simulink model "ARINC429_DW"  (R2020b)
settings: Solver=VariableStepAuto  StartTime=0.0  StopTime=10.0  RelTol=1e-3
(part 1 of 2)
settings Model: Creator=Nicolas  LastModifiedBy=rolla

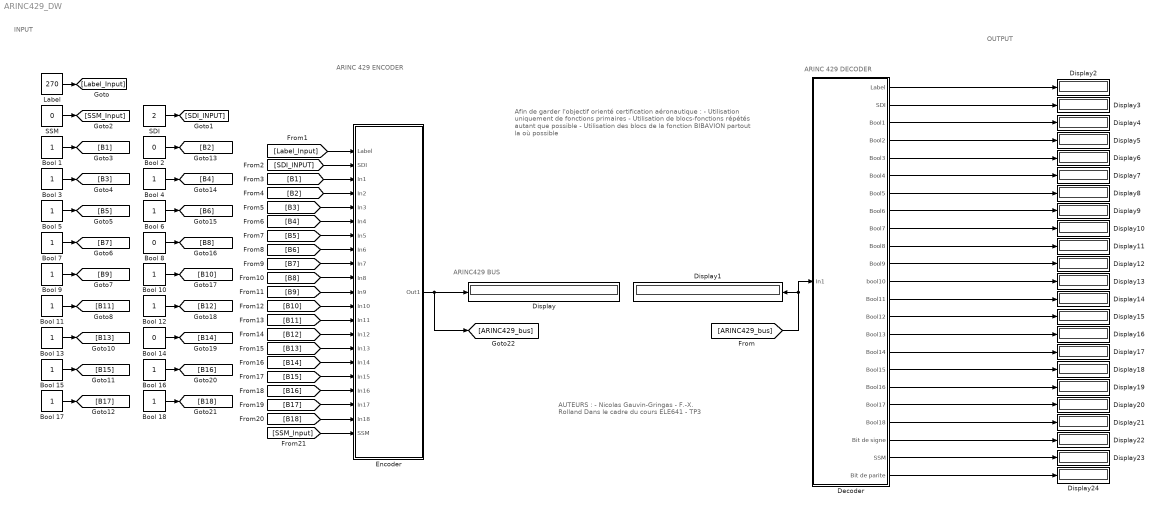
== system ARINC429_DW ==
  note: ARINC 429 DECODER
  note: ARINC 429 ENCODER
  note: ARINC429 BUS
  note: OUTPUT
  note: INPUT
  note: AUTEURS :
      | - Nicolas Gauvin-Gringas
      | - F.-X. Rolland
      |
      | Dans le cadre du cours ELE641 - TP3
  note: Afin de garder l'objectif orienté certification aéronautique :
      | - Utilisation uniquement de fonctions primaires
      | - Utilisation de blocs-fonctions répétés autant que possible
      | - Utilisation des blocs de la fonction BIBAVION partout la où possible
  Bool {1,3..7,9..13,15..18} (15 alike) : Constant  OutDataTypeStr=boolean
  Bool 14 : Constant  Value=0  OutDataTypeStr=boolean
  Bool 2 : Constant  Value=0  OutDataTypeStr=boolean
  Bool 8 : Constant  Value=0  OutDataTypeStr=boolean
  Decoder : Subsystem
  Display{,1..24} (25 alike) : Display
      Display settings: Format=binary (Stored Integer)
      Display1 settings: Format=binary (Stored Integer)
  Encoder : Subsystem
  Label : Constant  Value=270  OutDataTypeStr=uint32  SampleTime=-1
  SDI : Constant  Value=2  OutDataTypeStr=uint32  SampleTime=-1
  SSM : Constant  Value=0  OutDataTypeStr=uint32  SampleTime=-1
  wires:
  [ARINC429_bus] -> Decoder/1(In1), Display1/1
  Label/1 -> [Label_Input]
  SDI/1 -> [SDI_INPUT]
  SSM/1 -> [SSM_Input]
  Decoder/1(Label) -> Display2/1
  Bool 1/1 -> [B1]
  Bool 2/1 -> [B2]
  Bool 18/1 -> [B18]
  Bool 16/1 -> [B16]
  Bool 14/1 -> [B14]
  Bool 12/1 -> [B12]
  Bool 10/1 -> [B10]
  Bool 8/1 -> [B8]
  Bool 6/1 -> [B6]
  Bool 4/1 -> [B4]
  Bool 3/1 -> [B3]
  Bool 5/1 -> [B5]
  Bool 7/1 -> [B7]
  Bool 9/1 -> [B9]
  Bool 11/1 -> [B11]
  Bool 13/1 -> [B13]
  Bool 15/1 -> [B15]
  Bool 17/1 -> [B17]
  [Label_Input] -> Encoder/1(Label)
  Encoder/1(Out1) -> [ARINC429_bus], Display/1
  [SDI_INPUT] -> Encoder/2(SDI)
  [B1] -> Encoder/3(In1)
  [B2] -> Encoder/4(In2)
  [B3] -> Encoder/5(In3)
  [B4] -> Encoder/6(In4)
  [B5] -> Encoder/7(In5)
  [B6] -> Encoder/8(In6)
  [B7] -> Encoder/9(In7)
  [B8] -> Encoder/10(In8)
  [B9] -> Encoder/11(In9)
  [B10] -> Encoder/12(In10)
  [B11] -> Encoder/13(In11)
  [B12] -> Encoder/14(In12)
  [B13] -> Encoder/15(In13)
  [B14] -> Encoder/16(In14)
  [B15] -> Encoder/17(In15)
  [B16] -> Encoder/18(In16)
  [B17] -> Encoder/19(In17)
  [B18] -> Encoder/20(In18)
  [SSM_Input] -> Encoder/21(SSM)
  Decoder/2(SDI) -> Display3/1
  Decoder/3(Bool1) -> Display4/1
  Decoder/4(Bool2) -> Display5/1
  Decoder/5(Bool3) -> Display6/1
  Decoder/6(Bool4) -> Display7/1
  Decoder/7(Bool5) -> Display8/1
  Decoder/8(Bool6) -> Display9/1
  Decoder/9(Bool7) -> Display10/1
  Decoder/10(Bool8) -> Display11/1
  Decoder/11(Bool9) -> Display12/1
  Decoder/12(bool10) -> Display13/1
  Decoder/13(Bool11) -> Display14/1
  Decoder/14(Bool12) -> Display15/1
  Decoder/15(Bool13) -> Display16/1
  Decoder/16(Bool14) -> Display17/1
  Decoder/17(Bool15) -> Display18/1
  Decoder/18(Bool16) -> Display19/1
  Decoder/19(Bool17) -> Display20/1
  Decoder/20(Bool18) -> Display21/1
  Decoder/21(Bit de signe) -> Display22/1
  Decoder/22(SSM) -> Display23/1
  Decoder/23(Bit de parite) -> Display24/1

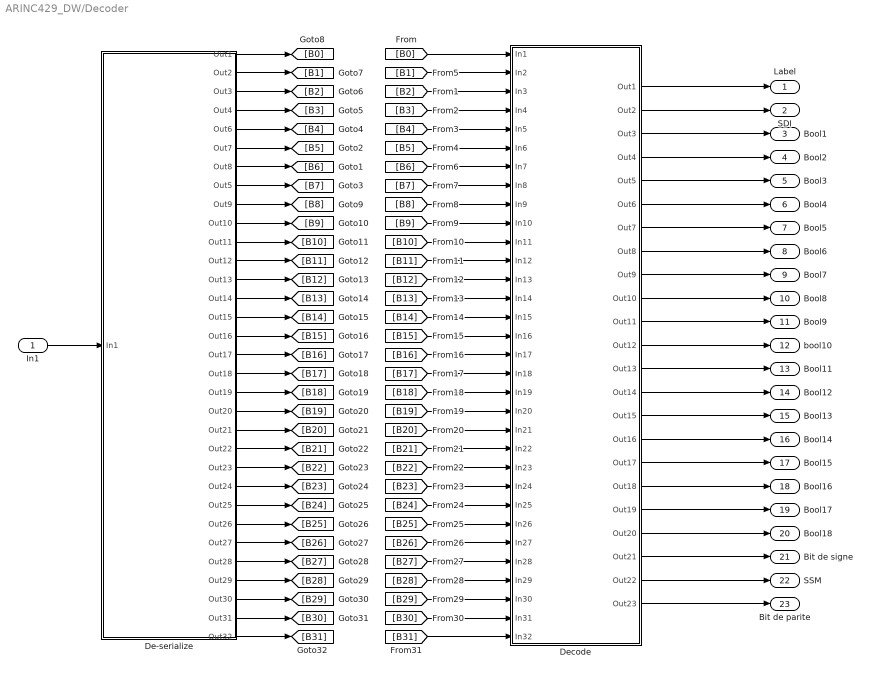
== system ARINC429_DW/Decoder ==
  In1 : Inport
  De-serialize : Subsystem
  Decode : Subsystem
  Label : Outport
  SDI : Outport  Port=2
  Bool1 : Outport  Port=3
  Bool2 : Outport  Port=4
  Bool3 : Outport  Port=5
  Bool4 : Outport  Port=6
  Bool5 : Outport  Port=7
  Bool6 : Outport  Port=8
  Bool7 : Outport  Port=9
  Bool8 : Outport  Port=10
  Bool9 : Outport  Port=11
  bool10 : Outport  Port=12
  Bool11 : Outport  Port=13
  Bool12 : Outport  Port=14
  Bool13 : Outport  Port=15
  Bool14 : Outport  Port=16
  Bool15 : Outport  Port=17
  Bool16 : Outport  Port=18
  Bool17 : Outport  Port=19
  Bool18 : Outport  Port=20
  Bit de signe : Outport  Port=21
  SSM : Outport  Port=22
  Bit de parite : Outport  Port=23
  wires:
  De-serialize/6(Out7) -> [B5]
  De-serialize/1(Out1) -> [B0]
  De-serialize/7(Out8) -> [B6]
  De-serialize/5(Out6) -> [B4]
  De-serialize/3(Out3) -> [B2]
  De-serialize/2(Out2) -> [B1]
  De-serialize/4(Out4) -> [B3]
  De-serialize/8(Out5) -> [B7]
  In1/1 -> De-serialize/1(In1)
  [B1] -> Decode/2(In2)
  [B0] -> Decode/1(In1)
  [B2] -> Decode/3(In3)
  [B3] -> Decode/4(In4)
  [B4] -> Decode/5(In5)
  [B5] -> Decode/6(In6)
  [B6] -> Decode/7(In7)
  [B7] -> Decode/8(In8)
  Decode/1(Out1) -> Label/1
  De-serialize/9(Out9) -> [B8]
  De-serialize/10(Out10) -> [B9]
  De-serialize/11(Out11) -> [B10]
  De-serialize/12(Out12) -> [B11]
  De-serialize/13(Out13) -> [B12]
  De-serialize/14(Out14) -> [B13]
  De-serialize/15(Out15) -> [B14]
  De-serialize/16(Out16) -> [B15]
  De-serialize/17(Out17) -> [B16]
  De-serialize/18(Out18) -> [B17]
  De-serialize/19(Out19) -> [B18]
  De-serialize/20(Out20) -> [B19]
  De-serialize/21(Out21) -> [B20]
  De-serialize/22(Out22) -> [B21]
  De-serialize/23(Out23) -> [B22]
  De-serialize/24(Out24) -> [B23]
  De-serialize/25(Out25) -> [B24]
  De-serialize/26(Out26) -> [B25]
  De-serialize/27(Out27) -> [B26]
  De-serialize/28(Out28) -> [B27]
  De-serialize/29(Out29) -> [B28]
  De-serialize/30(Out30) -> [B29]
  De-serialize/31(Out31) -> [B30]
  De-serialize/32(Out32) -> [B31]
  [B8] -> Decode/9(In9)
  [B9] -> Decode/10(In10)
  [B10] -> Decode/11(In11)
  [B11] -> Decode/12(In12)
  [B12] -> Decode/13(In13)
  [B13] -> Decode/14(In14)
  [B14] -> Decode/15(In15)
  [B15] -> Decode/16(In16)
  [B16] -> Decode/17(In17)
  [B17] -> Decode/18(In18)
  [B18] -> Decode/19(In19)
  [B19] -> Decode/20(In20)
  [B20] -> Decode/21(In21)
  [B21] -> Decode/22(In22)
  [B22] -> Decode/23(In23)
  [B23] -> Decode/24(In24)
  [B24] -> Decode/25(In25)
  [B25] -> Decode/26(In26)
  [B26] -> Decode/27(In27)
  [B27] -> Decode/28(In28)
  [B28] -> Decode/29(In29)
  [B29] -> Decode/30(In30)
  [B30] -> Decode/31(In31)
  [B31] -> Decode/32(In32)
  Decode/3(Out3) -> Bool1/1
  Decode/4(Out4) -> Bool2/1
  Decode/5(Out5) -> Bool3/1
  Decode/10(Out10) -> Bool8/1
  Decode/11(Out11) -> Bool9/1
  Decode/12(Out12) -> bool10/1
  Decode/13(Out13) -> Bool11/1
  Decode/14(Out14) -> Bool12/1
  Decode/15(Out15) -> Bool13/1
  Decode/16(Out16) -> Bool14/1
  Decode/17(Out17) -> Bool15/1
  Decode/18(Out18) -> Bool16/1
  Decode/19(Out19) -> Bool17/1
  Decode/20(Out20) -> Bool18/1
  Decode/21(Out21) -> Bit de signe/1
  Decode/22(Out22) -> SSM/1
  Decode/23(Out23) -> Bit de parite/1
  Decode/9(Out9) -> Bool7/1
  Decode/8(Out8) -> Bool6/1
  Decode/7(Out7) -> Bool5/1
  Decode/6(Out6) -> Bool4/1
  Decode/2(Out2) -> SDI/1

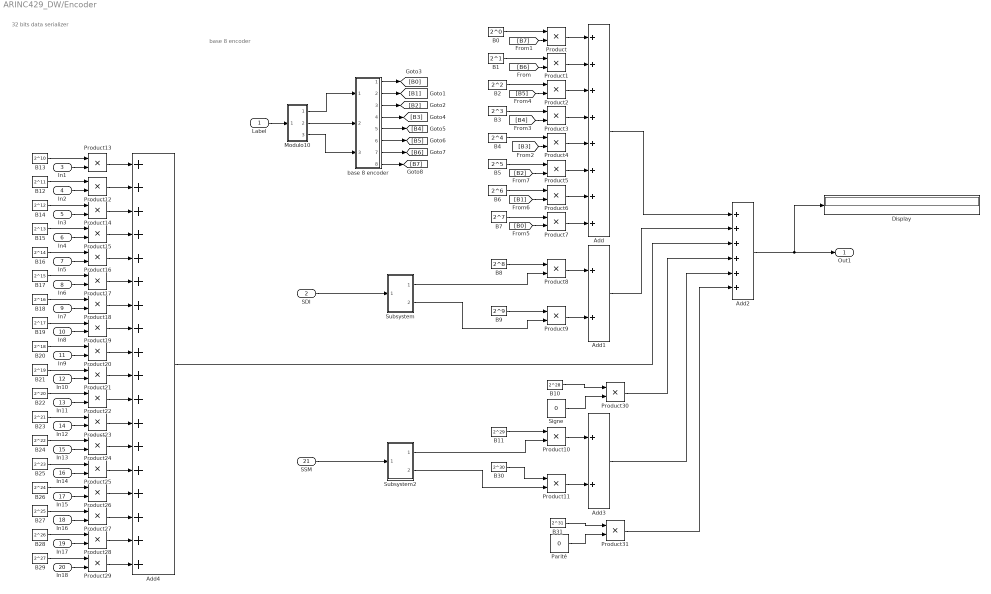
== system ARINC429_DW/Encoder ==
  note: base 8 encoder
  note: 32 bits data serializer
  Label : Inport
  SDI : Inport  Port=2
  In1 : Inport  Port=3
  In2 : Inport  Port=4
  In3 : Inport  Port=5
  In4 : Inport  Port=6
  In5 : Inport  Port=7
  In6 : Inport  Port=8
  In7 : Inport  Port=9
  In8 : Inport  Port=10
  In9 : Inport  Port=11
  In10 : Inport  Port=12
  In11 : Inport  Port=13
  In12 : Inport  Port=14
  In13 : Inport  Port=15
  In14 : Inport  Port=16
  In15 : Inport  Port=17
  In16 : Inport  Port=18
  In17 : Inport  Port=19
  In18 : Inport  Port=20
  SSM : Inport  Port=21
  Add : Sum  Inputs=++++++++  AccumDataTypeStr=uint32  OutDataTypeStr=uint32
  Add1 : Sum
  Add2 : Sum  Inputs=++++++  AccumDataTypeStr=uint32  OutDataTypeStr=uint32
  Add3 : Sum
  Add4 : Sum  Inputs=++++++++++++++++++
  B0 : Constant  Value=2^0  OutDataTypeStr=single
  B1 : Constant  Value=2^1  OutDataTypeStr=single
  B10 : Constant  Value=2^28  OutDataTypeStr=single
  B11 : Constant  Value=2^29  OutDataTypeStr=single
  B12 : Constant  Value=2^11  OutDataTypeStr=single
  B13 : Constant  Value=2^10  OutDataTypeStr=single
  B14 : Constant  Value=2^12  OutDataTypeStr=single
  B15 : Constant  Value=2^13  OutDataTypeStr=single
  B16 : Constant  Value=2^14  OutDataTypeStr=single
  B17 : Constant  Value=2^15  OutDataTypeStr=single
  B18 : Constant  Value=2^16  OutDataTypeStr=single
  B19 : Constant  Value=2^17  OutDataTypeStr=single
  B2 : Constant  Value=2^2  OutDataTypeStr=single
  B20 : Constant  Value=2^18  OutDataTypeStr=single
  B21 : Constant  Value=2^19  OutDataTypeStr=single
  B22 : Constant  Value=2^20  OutDataTypeStr=single
  B23 : Constant  Value=2^21  OutDataTypeStr=single
  B24 : Constant  Value=2^22  OutDataTypeStr=single
  B25 : Constant  Value=2^23  OutDataTypeStr=single
  B26 : Constant  Value=2^24  OutDataTypeStr=single
  B27 : Constant  Value=2^25  OutDataTypeStr=single
  B28 : Constant  Value=2^26  OutDataTypeStr=single
  B29 : Constant  Value=2^27  OutDataTypeStr=single
  B3 : Constant  Value=2^3  OutDataTypeStr=single
  B30 : Constant  Value=2^30  OutDataTypeStr=single
  B31 : Constant  Value=2^31  OutDataTypeStr=single
  B4 : Constant  Value=2^4  OutDataTypeStr=single
  B5 : Constant  Value=2^5  OutDataTypeStr=single
  B6 : Constant  Value=2^6  OutDataTypeStr=single
  B7 : Constant  Value=2^7  OutDataTypeStr=single
  B8 : Constant  Value=2^8  OutDataTypeStr=single
  B9 : Constant  Value=2^9  OutDataTypeStr=single
  Display : Display
      settings: Format=binary (Stored Integer)
  "Modulo10 " : Subsystem
  Parité : Constant  Value=0  OutDataTypeStr=boolean
  Product{,1..31} (32 alike) : Product
  Signe : Constant  Value=0  OutDataTypeStr=boolean
  Subsystem : Subsystem
  Subsystem2 : Subsystem
  base 8 encoder : Subsystem
  Out1 : Outport
  wires:
  base 8 encoder/4(Out4) -> [B3]
  B5/1 -> Product5/1
  [B0] -> Product7/2
  B2/1 -> Product2/1
  [B5] -> Product2/2
  [B3] -> Product4/2
  "Modulo10 "/2(Out2) -> base 8 encoder/2(In2)
  "Modulo10 "/3(Out3) -> base 8 encoder/3(In3)
  B0/1 -> Product/1
  Product3/1 -> Add/4
  [B7] -> Product/2
  Product4/1 -> Add/5
  base 8 encoder/5(Out5) -> [B4]
  base 8 encoder/8(Out8) -> [B7]
  [B6] -> Product1/2
  B1/1 -> Product1/1
  [B4] -> Product3/2
  B4/1 -> Product4/1
  base 8 encoder/3(Out3) -> [B2]
  Product/1 -> Add/1
  Product5/1 -> Add/6
  Product6/1 -> Add/7
  base 8 encoder/1(Out1) -> [B0]
  [B1] -> Product6/2
  base 8 encoder/7(Out7) -> [B6]
  Product2/1 -> Add/3
  B3/1 -> Product3/1
  Label/1 -> "Modulo10 "/1(In1)
  Product7/1 -> Add/8
  Product1/1 -> Add/2
  B6/1 -> Product6/1
  B7/1 -> Product7/1
  "Modulo10 "/1(Out1) -> base 8 encoder/1(In1)
  base 8 encoder/6(Out6) -> [B5]
  [B2] -> Product5/2
  base 8 encoder/2(Out2) -> [B1]
  Product9/1 -> Add1/2
  Product8/1 -> Add1/1
  B9/1 -> Product9/1
  B8/1 -> Product8/1
  Product10/1 -> Add3/1
  Product11/1 -> Add3/2
  B13/1 -> Product13/1
  Product13/1 -> Add4/1
  B12/1 -> Product12/1
  Product12/1 -> Add4/2
  B14/1 -> Product14/1
  Product14/1 -> Add4/3
  B15/1 -> Product15/1
  Product15/1 -> Add4/4
  B16/1 -> Product16/1
  Product16/1 -> Add4/5
  B17/1 -> Product17/1
  Product17/1 -> Add4/6
  B18/1 -> Product18/1
  Product18/1 -> Add4/7
  B19/1 -> Product19/1
  Product19/1 -> Add4/8
  B20/1 -> Product20/1
  Product20/1 -> Add4/9
  B21/1 -> Product21/1
  Product21/1 -> Add4/10
  B22/1 -> Product22/1
  Product22/1 -> Add4/11
  B23/1 -> Product23/1
  Product23/1 -> Add4/12
  B24/1 -> Product24/1
  Product24/1 -> Add4/13
  B25/1 -> Product25/1
  Product25/1 -> Add4/14
  B26/1 -> Product26/1
  Product26/1 -> Add4/15
  B27/1 -> Product27/1
  Product27/1 -> Add4/16
  B28/1 -> Product28/1
  Product28/1 -> Add4/17
  B29/1 -> Product29/1
  Product29/1 -> Add4/18
  In1/1 -> Product13/2
  In2/1 -> Product12/2
  In3/1 -> Product14/2
  In4/1 -> Product15/2
  In5/1 -> Product16/2
  In6/1 -> Product17/2
  In7/1 -> Product18/2
  In8/1 -> Product19/2
  In9/1 -> Product20/2
  In10/1 -> Product21/2
  In11/1 -> Product22/2
  In12/1 -> Product23/2
  In13/1 -> Product24/2
  In14/1 -> Product25/2
  In15/1 -> Product26/2
  In16/1 -> Product27/2
  In17/1 -> Product28/2
  In18/1 -> Product29/2
  SDI/1 -> Subsystem/1(In1)
  Subsystem/1(Out1) -> Product8/2
  Subsystem/2(Out2) -> Product9/2
  SSM/1 -> Subsystem2/1(In1)
  Subsystem2/1(Out1) -> Product10/2
  Subsystem2/2(Out2) -> Product11/2
  Signe/1 -> Product30/2
  B31/1 -> Product31/1
  Parité/1 -> Product31/2
  B11/1 -> Product10/1
  B10/1 -> Product30/1
  Add2/1 -> Display/1, Out1/1
  Add/1 -> Add2/1
  Add1/1 -> Add2/2
  Add4/1 -> Add2/3
  Product30/1 -> Add2/4
  Add3/1 -> Add2/5
  Product31/1 -> Add2/6
  B30/1 -> Product11/1

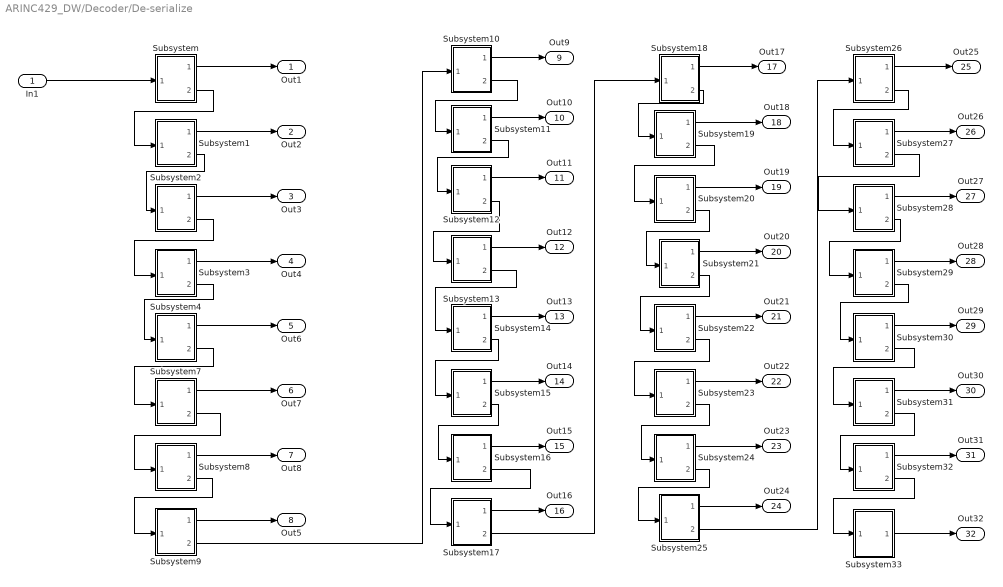
== system ARINC429_DW/Decoder/De-serialize ==
  In1 : Inport
  Subsystem : Subsystem
  Subsystem1 : Subsystem
  Subsystem10 : Subsystem
  Subsystem11 : Subsystem
  Subsystem12 : Subsystem
  Subsystem13 : Subsystem
  Subsystem14 : Subsystem
  Subsystem15 : Subsystem
  Subsystem16 : Subsystem
  Subsystem17 : Subsystem
  Subsystem18 : Subsystem
  Subsystem19 : Subsystem
  Subsystem2 : Subsystem
  Subsystem20 : Subsystem
  Subsystem21 : Subsystem
  Subsystem22 : Subsystem
  Subsystem23 : Subsystem
  Subsystem24 : Subsystem
  Subsystem25 : Subsystem
  Subsystem26 : Subsystem
  Subsystem27 : Subsystem
  Subsystem28 : Subsystem
  Subsystem29 : Subsystem
  Subsystem3 : Subsystem
  Subsystem30 : Subsystem
  Subsystem31 : Subsystem
  Subsystem32 : Subsystem
  Subsystem33 : Subsystem
  Subsystem4 : Subsystem
  Subsystem7 : Subsystem
  Subsystem8 : Subsystem
  Subsystem9 : Subsystem
  Out1 : Outport
  Out2 : Outport  Port=2
  Out3 : Outport  Port=3
  Out4 : Outport  Port=4
  Out6 : Outport  Port=5
  Out7 : Outport  Port=6
  Out8 : Outport  Port=7
  Out5 : Outport  Port=8
  Out9 : Outport  Port=9
  Out10 : Outport  Port=10
  Out11 : Outport  Port=11
  Out12 : Outport  Port=12
  Out13 : Outport  Port=13
  Out14 : Outport  Port=14
  Out15 : Outport  Port=15
  Out16 : Outport  Port=16
  Out17 : Outport  Port=17
  Out18 : Outport  Port=18
  Out19 : Outport  Port=19
  Out20 : Outport  Port=20
  Out21 : Outport  Port=21
  Out22 : Outport  Port=22
  Out23 : Outport  Port=23
  Out24 : Outport  Port=24
  Out25 : Outport  Port=25
  Out26 : Outport  Port=26
  Out27 : Outport  Port=27
  Out28 : Outport  Port=28
  Out29 : Outport  Port=29
  Out30 : Outport  Port=30
  Out31 : Outport  Port=31
  Out32 : Outport  Port=32
  wires:
  Subsystem/1(Out1) -> Out1/1
  Subsystem1/1(Out1) -> Out2/1
  Subsystem1/2(Out2) -> Subsystem2/1(In1)
  Subsystem2/2(Out2) -> Subsystem3/1(In1)
  Subsystem3/2(Out2) -> Subsystem4/1(In1)
  Subsystem2/1(Out1) -> Out3/1
  Subsystem3/1(Out1) -> Out4/1
  Subsystem4/2(Out2) -> Subsystem7/1(In1)
  Subsystem4/1(Out1) -> Out6/1
  Subsystem7/1(Out1) -> Out7/1
  Subsystem8/1(Out1) -> Out8/1
  Subsystem10/2(Out2) -> Subsystem11/1(In1)
  Subsystem12/2(Out2) -> Subsystem13/1(In1)
  Subsystem14/2(Out2) -> Subsystem15/1(In1)
  Subsystem11/2(Out2) -> Subsystem12/1(In1)
  Subsystem15/2(Out2) -> Subsystem16/1(In1)
  Subsystem16/2(Out2) -> Subsystem17/1(In1)
  Subsystem23/2(Out2) -> Subsystem24/1(In1)
  Subsystem18/2(Out2) -> Subsystem19/1(In1)
  Subsystem21/2(Out2) -> Subsystem22/1(In1)
  Subsystem22/2(Out2) -> Subsystem23/1(In1)
  Subsystem19/2(Out2) -> Subsystem20/1(In1)
  Subsystem20/2(Out2) -> Subsystem21/1(In1)
  Subsystem24/2(Out2) -> Subsystem25/1(In1)
  Subsystem29/2(Out2) -> Subsystem30/1(In1)
  Subsystem27/2(Out2) -> Subsystem28/1(In1)
  Subsystem28/2(Out2) -> Subsystem29/1(In1)
  Subsystem26/2(Out2) -> Subsystem27/1(In1)
  Subsystem9/1(Out1) -> Out5/1
  Subsystem17/2(Out2) -> Subsystem18/1(In1)
  Subsystem25/2(Out2) -> Subsystem26/1(In1)
  Subsystem9/2(Out2) -> Subsystem10/1(In1)
  Subsystem10/1(Out1) -> Out9/1
  Subsystem11/1(Out1) -> Out10/1
  Subsystem12/1(Out1) -> Out11/1
  Subsystem13/1(Out1) -> Out12/1
  Subsystem14/1(Out1) -> Out13/1
  Subsystem15/1(Out1) -> Out14/1
  Subsystem16/1(Out1) -> Out15/1
  Subsystem17/1(Out1) -> Out16/1
  Subsystem18/1(Out1) -> Out17/1
  Subsystem19/1(Out1) -> Out18/1
  Subsystem20/1(Out1) -> Out19/1
  Subsystem21/1(Out1) -> Out20/1
  Subsystem22/1(Out1) -> Out21/1
  Subsystem23/1(Out1) -> Out22/1
  Subsystem24/1(Out1) -> Out23/1
  Subsystem25/1(Out1) -> Out24/1
  Subsystem26/1(Out1) -> Out25/1
  Subsystem27/1(Out1) -> Out26/1
  Subsystem28/1(Out1) -> Out27/1
  Subsystem29/1(Out1) -> Out28/1
  Subsystem33/1(Out1) -> Out32/1
  Subsystem30/2(Out2) -> Subsystem31/1(In1)
  Subsystem31/2(Out2) -> Subsystem32/1(In1)
  Subsystem32/2(Out2) -> Subsystem33/1(In1)
  Subsystem32/1(Out1) -> Out31/1
  Subsystem31/1(Out1) -> Out30/1
  Subsystem30/1(Out1) -> Out29/1
  Subsystem7/2(Out2) -> Subsystem8/1(In1)
  Subsystem8/2(Out2) -> Subsystem9/1(In1)
  Subsystem/2(Out2) -> Subsystem1/1(In1)
  In1/1 -> Subsystem/1(In1)
  Subsystem13/2(Out2) -> Subsystem14/1(In1)

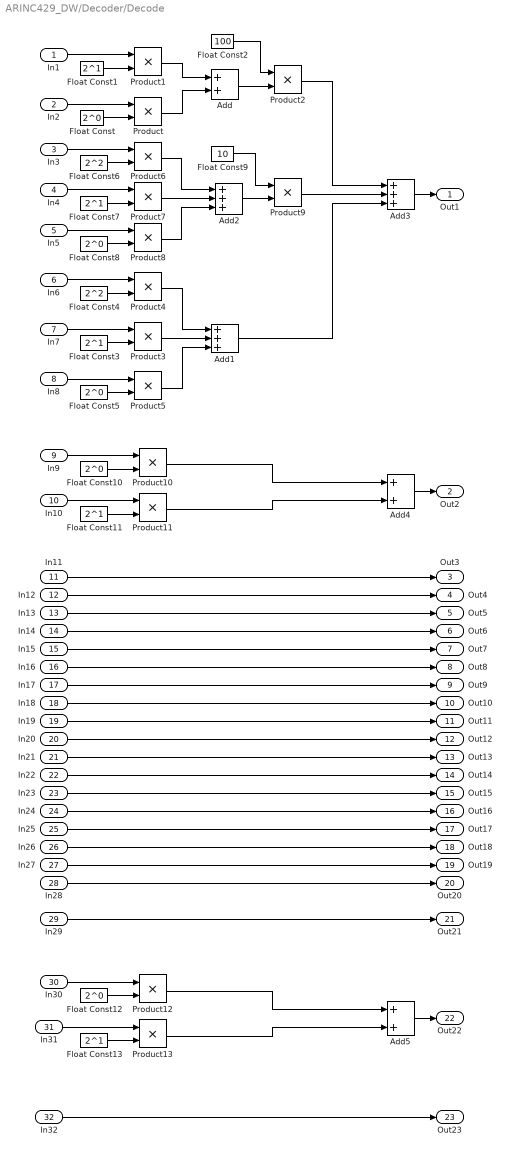
== system ARINC429_DW/Decoder/Decode ==
  In1 : Inport
  In2 : Inport  Port=2
  In3 : Inport  Port=3
  In4 : Inport  Port=4
  In5 : Inport  Port=5
  In6 : Inport  Port=6
  In7 : Inport  Port=7
  In8 : Inport  Port=8
  In9 : Inport  Port=9
  In10 : Inport  Port=10
  In11 : Inport  Port=11
  In12 : Inport  Port=12
  In13 : Inport  Port=13
  In14 : Inport  Port=14
  In15 : Inport  Port=15
  In16 : Inport  Port=16
  In17 : Inport  Port=17
  In18 : Inport  Port=18
  In19 : Inport  Port=19
  In20 : Inport  Port=20
  In21 : Inport  Port=21
  In22 : Inport  Port=22
  In23 : Inport  Port=23
  In24 : Inport  Port=24
  In25 : Inport  Port=25
  In26 : Inport  Port=26
  In27 : Inport  Port=27
  In28 : Inport  Port=28
  In29 : Inport  Port=29
  In30 : Inport  Port=30
  In31 : Inport  Port=31
  In32 : Inport  Port=32
  Add : Sum
  Add1 : Sum  Inputs=+++
  Add2 : Sum  Inputs=+++
  Add3 : Sum  Inputs=+++
  Add4 : Sum
  Add5 : Sum
  Float Const{,5,8,10,12} (5 alike) : Constant  Value=2^0  OutDataTypeStr=single
  Float Const{1,3,7,11,13} (5 alike) : Constant  Value=2^1  OutDataTypeStr=single
  Float Const2 : Constant  Value=100  OutDataTypeStr=single
  Float Const4 : Constant  Value=2^2  OutDataTypeStr=single
  Float Const6 : Constant  Value=2^2  OutDataTypeStr=single
  Float Const9 : Constant  Value=10  OutDataTypeStr=single
  Product{,1..13} (14 alike) : Product
  Out1 : Outport
  Out2 : Outport  Port=2
  Out3 : Outport  Port=3
  Out4 : Outport  Port=4
  Out5 : Outport  Port=5
  Out6 : Outport  Port=6
  Out7 : Outport  Port=7
  Out8 : Outport  Port=8
  Out9 : Outport  Port=9
  Out10 : Outport  Port=10
  Out11 : Outport  Port=11
  Out12 : Outport  Port=12
  Out13 : Outport  Port=13
  Out14 : Outport  Port=14
  Out15 : Outport  Port=15
  Out16 : Outport  Port=16
  Out17 : Outport  Port=17
  Out18 : Outport  Port=18
  Out19 : Outport  Port=19
  Out20 : Outport  Port=20
  Out21 : Outport  Port=21
  Out22 : Outport  Port=22
  Out23 : Outport  Port=23
  wires:
  Float Const6/1 -> Product6/2
  In5/1 -> Product8/1
  Product/1 -> Add/2
  Float Const5/1 -> Product5/2
  Float Const3/1 -> Product3/2
  Product6/1 -> Add2/1
  In6/1 -> Product4/1
  Product3/1 -> Add1/2
  In8/1 -> Product5/1
  Product7/1 -> Add2/2
  Product8/1 -> Add2/3
  Product1/1 -> Add/1
  Product4/1 -> Add1/1
  Float Const8/1 -> Product8/2
  Float Const1/1 -> Product1/2
  Product5/1 -> Add1/3
  In3/1 -> Product6/1
  Float Const/1 -> Product/2
  Float Const4/1 -> Product4/2
  Float Const7/1 -> Product7/2
  In1/1 -> Product1/1
  In2/1 -> Product/1
  In7/1 -> Product3/1
  In4/1 -> Product7/1
  Add2/1 -> Product9/2
  Add/1 -> Product2/2
  Float Const2/1 -> Product2/1
  Float Const9/1 -> Product9/1
  Add1/1 -> Add3/3
  Product9/1 -> Add3/2
  Add3/1 -> Out1/1
  Float Const10/1 -> Product10/2
  In9/1 -> Product10/1
  Float Const11/1 -> Product11/2
  In10/1 -> Product11/1
  Product10/1 -> Add4/1
  Product11/1 -> Add4/2
  Add4/1 -> Out2/1
  Product12/1 -> Add5/1
  In31/1 -> Product13/1
  Product13/1 -> Add5/2
  Float Const13/1 -> Product13/2
  Float Const12/1 -> Product12/2
  Add5/1 -> Out22/1
  In30/1 -> Product12/1
  In32/1 -> Out23/1
  In29/1 -> Out21/1
  In28/1 -> Out20/1
  In27/1 -> Out19/1
  In26/1 -> Out18/1
  In11/1 -> Out3/1
  In12/1 -> Out4/1
  In13/1 -> Out5/1
  In14/1 -> Out6/1
  In15/1 -> Out7/1
  In16/1 -> Out8/1
  In17/1 -> Out9/1
  In18/1 -> Out10/1
  In19/1 -> Out11/1
  In20/1 -> Out12/1
  In21/1 -> Out13/1
  In22/1 -> Out14/1
  In23/1 -> Out15/1
  In24/1 -> Out16/1
  In25/1 -> Out17/1
  Product2/1 -> Add3/1

== system ARINC429_DW/Encoder/Modulo10  ==
  In1 : Inport
  Subsystem : Subsystem
  Subsystem1 : Subsystem
  Subsystem2 : Subsystem
  Out1 : Outport
  Out2 : Outport  Port=2
  Out3 : Outport  Port=3
  wires:
  In1/1 -> Subsystem/1(In1)
  Subsystem/1(Out1) -> Out1/1
  Subsystem/2(Out2) -> Subsystem1/1(In1)
  Subsystem1/1(Out1) -> Out2/1
  Subsystem1/2(Out2) -> Subsystem2/1(In1)
  Subsystem2/1(Out1) -> Out3/1

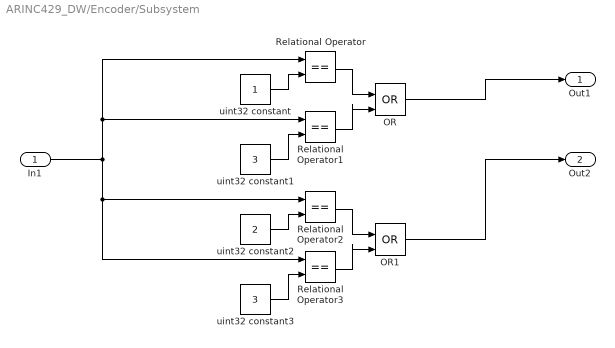
== system ARINC429_DW/Encoder/Subsystem ==
  In1 : Inport
  OR : Logic  Operator=OR  IconShape=distinctive  AllPortsSameDT=off  OutDataTypeStr=boolean
  OR1 : Logic  Operator=OR  IconShape=distinctive  AllPortsSameDT=off  OutDataTypeStr=boolean
  Relational Operator{,1..3} (4 alike) : RelationalOperator  Operator===  OutDataTypeStr=boolean  RndMeth=Nearest
  uint32 constant : Constant  OutDataTypeStr=uint32  SampleTime=-1
  uint32 constant1 : Constant  Value=3  OutDataTypeStr=uint32  SampleTime=-1
  uint32 constant2 : Constant  Value=2  OutDataTypeStr=uint32  SampleTime=-1
  uint32 constant3 : Constant  Value=3  OutDataTypeStr=uint32  SampleTime=-1
  Out1 : Outport
  Out2 : Outport  Port=2
  wires:
  uint32 constant1/1 -> Relational Operator1/2
  Relational Operator1/1 -> OR/2
  uint32 constant3/1 -> Relational Operator3/2
  Relational Operator/1 -> OR/1
  uint32 constant2/1 -> Relational Operator2/2
  In1/1 -> Relational Operator/1, Relational Operator1/1, Relational Operator3/1, Relational Operator2/1
  Relational Operator3/1 -> OR1/2
  uint32 constant/1 -> Relational Operator/2
  Relational Operator2/1 -> OR1/1
  OR1/1 -> Out2/1
  OR/1 -> Out1/1

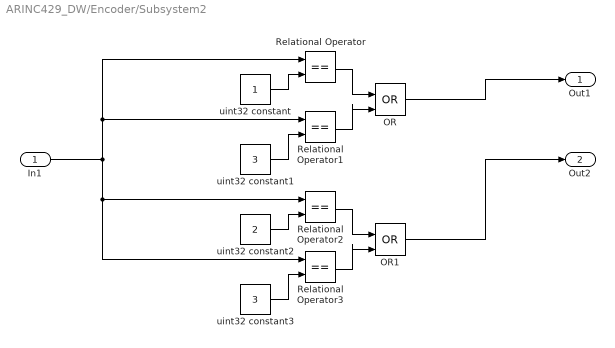
== system ARINC429_DW/Encoder/Subsystem2 ==
  In1 : Inport
  OR : Logic  Operator=OR  IconShape=distinctive  AllPortsSameDT=off  OutDataTypeStr=boolean
  OR1 : Logic  Operator=OR  IconShape=distinctive  AllPortsSameDT=off  OutDataTypeStr=boolean
  Relational Operator{,1..3} (4 alike) : RelationalOperator  Operator===  OutDataTypeStr=boolean  RndMeth=Nearest
  uint32 constant : Constant  OutDataTypeStr=uint32  SampleTime=-1
  uint32 constant1 : Constant  Value=3  OutDataTypeStr=uint32  SampleTime=-1
  uint32 constant2 : Constant  Value=2  OutDataTypeStr=uint32  SampleTime=-1
  uint32 constant3 : Constant  Value=3  OutDataTypeStr=uint32  SampleTime=-1
  Out1 : Outport
  Out2 : Outport  Port=2
  wires:
  uint32 constant1/1 -> Relational Operator1/2
  Relational Operator1/1 -> OR/2
  uint32 constant3/1 -> Relational Operator3/2
  Relational Operator/1 -> OR/1
  uint32 constant2/1 -> Relational Operator2/2
  In1/1 -> Relational Operator/1, Relational Operator1/1, Relational Operator3/1, Relational Operator2/1
  Relational Operator3/1 -> OR1/2
  uint32 constant/1 -> Relational Operator/2
  Relational Operator2/1 -> OR1/1
  OR1/1 -> Out2/1
  OR/1 -> Out1/1

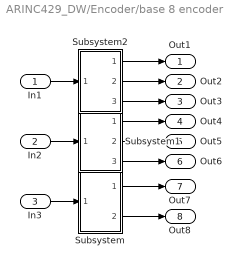
== system ARINC429_DW/Encoder/base 8 encoder ==
  In1 : Inport
  In2 : Inport  Port=2
  In3 : Inport  Port=3
  Subsystem : Subsystem
  Subsystem1 : Subsystem
  Subsystem2 : Subsystem
  Out1 : Outport
  Out2 : Outport  Port=2
  Out3 : Outport  Port=3
  Out4 : Outport  Port=4
  Out5 : Outport  Port=5
  Out6 : Outport  Port=6
  Out7 : Outport  Port=7
  Out8 : Outport  Port=8
  wires:
  In2/1 -> Subsystem1/1(In1)
  In1/1 -> Subsystem2/1(In1)
  In3/1 -> Subsystem/1(In1)
  Subsystem2/1(Out1) -> Out1/1
  Subsystem2/2(Out2) -> Out2/1
  Subsystem1/1(Out1) -> Out4/1
  Subsystem1/2(Out2) -> Out5/1
  Subsystem1/3(Out3) -> Out6/1
  Subsystem/1(Out1) -> Out7/1
  Subsystem/2(Out2) -> Out8/1
  Subsystem2/3(Out3) -> Out3/1

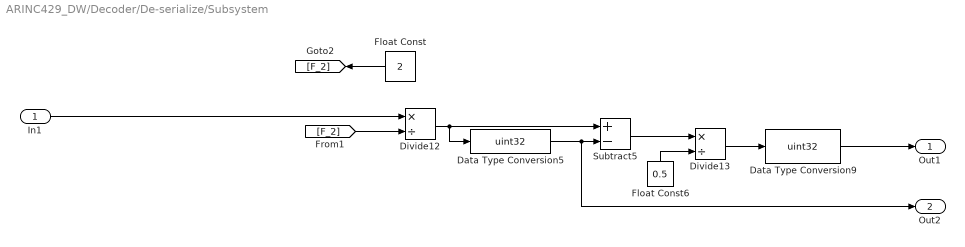
== system ARINC429_DW/Decoder/De-serialize/Subsystem ==
  In1 : Inport
  Data Type Conversion5 : DataTypeConversion  OutDataTypeStr=uint32
  Data Type Conversion9 : DataTypeConversion  OutDataTypeStr=uint32
  Divide12 : Product  Inputs=*/  OutDataTypeStr=double
  Divide13 : Product  Inputs=*/  OutDataTypeStr=uint32
  Float Const : Constant  Value=2  OutDataTypeStr=single
  Float Const6 : Constant  Value=0.5  OutDataTypeStr=single
  Subtract5 : Sum  Inputs=+-
  Out1 : Outport
  Out2 : Outport  Port=2
  wires:
  Float Const/1 -> [F_2]
  Divide12/1 -> Subtract5/1, Data Type Conversion5/1
  Divide13/1 -> Data Type Conversion9/1
  Float Const6/1 -> Divide13/2
  Data Type Conversion5/1 -> Out2/1, Subtract5/2
  [F_2] -> Divide12/2
  Subtract5/1 -> Divide13/1
  Data Type Conversion9/1 -> Out1/1
  In1/1 -> Divide12/1

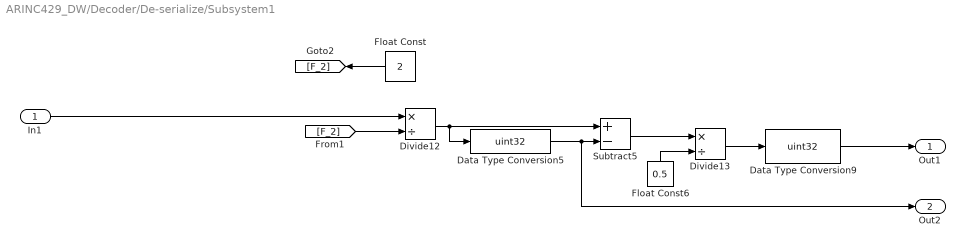
== system ARINC429_DW/Decoder/De-serialize/Subsystem1 ==
  In1 : Inport
  Data Type Conversion5 : DataTypeConversion  OutDataTypeStr=uint32
  Data Type Conversion9 : DataTypeConversion  OutDataTypeStr=uint32
  Divide12 : Product  Inputs=*/  OutDataTypeStr=double
  Divide13 : Product  Inputs=*/  OutDataTypeStr=uint32
  Float Const : Constant  Value=2  OutDataTypeStr=single
  Float Const6 : Constant  Value=0.5  OutDataTypeStr=single
  Subtract5 : Sum  Inputs=+-
  Out1 : Outport
  Out2 : Outport  Port=2
  wires:
  Float Const/1 -> [F_2]
  Divide12/1 -> Subtract5/1, Data Type Conversion5/1
  Divide13/1 -> Data Type Conversion9/1
  Float Const6/1 -> Divide13/2
  Data Type Conversion5/1 -> Out2/1, Subtract5/2
  [F_2] -> Divide12/2
  Subtract5/1 -> Divide13/1
  Data Type Conversion9/1 -> Out1/1
  In1/1 -> Divide12/1

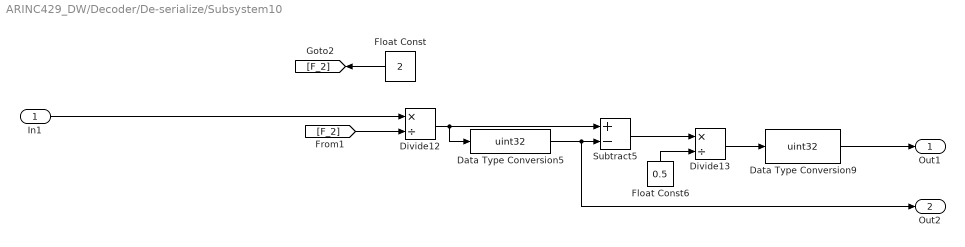
== system ARINC429_DW/Decoder/De-serialize/Subsystem10 ==
  In1 : Inport
  Data Type Conversion5 : DataTypeConversion  OutDataTypeStr=uint32
  Data Type Conversion9 : DataTypeConversion  OutDataTypeStr=uint32
  Divide12 : Product  Inputs=*/  OutDataTypeStr=double
  Divide13 : Product  Inputs=*/  OutDataTypeStr=uint32
  Float Const : Constant  Value=2  OutDataTypeStr=single
  Float Const6 : Constant  Value=0.5  OutDataTypeStr=single
  Subtract5 : Sum  Inputs=+-
  Out1 : Outport
  Out2 : Outport  Port=2
  wires:
  Float Const/1 -> [F_2]
  Divide12/1 -> Subtract5/1, Data Type Conversion5/1
  Divide13/1 -> Data Type Conversion9/1
  Float Const6/1 -> Divide13/2
  Data Type Conversion5/1 -> Out2/1, Subtract5/2
  [F_2] -> Divide12/2
  Subtract5/1 -> Divide13/1
  Data Type Conversion9/1 -> Out1/1
  In1/1 -> Divide12/1

== system ARINC429_DW/Decoder/De-serialize/Subsystem11 ==
  In1 : Inport
  Data Type Conversion5 : DataTypeConversion  OutDataTypeStr=uint32
  Data Type Conversion9 : DataTypeConversion  OutDataTypeStr=uint32
  Divide12 : Product  Inputs=*/  OutDataTypeStr=double
  Divide13 : Product  Inputs=*/  OutDataTypeStr=uint32
  Float Const : Constant  Value=2  OutDataTypeStr=single
  Float Const6 : Constant  Value=0.5  OutDataTypeStr=single
  Subtract5 : Sum  Inputs=+-
  Out1 : Outport
  Out2 : Outport  Port=2
  wires:
  Float Const/1 -> [F_2]
  Divide12/1 -> Subtract5/1, Data Type Conversion5/1
  Divide13/1 -> Data Type Conversion9/1
  Float Const6/1 -> Divide13/2
  Data Type Conversion5/1 -> Out2/1, Subtract5/2
  [F_2] -> Divide12/2
  Subtract5/1 -> Divide13/1
  Data Type Conversion9/1 -> Out1/1
  In1/1 -> Divide12/1

== system ARINC429_DW/Decoder/De-serialize/Subsystem12 ==
  In1 : Inport
  Data Type Conversion5 : DataTypeConversion  OutDataTypeStr=uint32
  Data Type Conversion9 : DataTypeConversion  OutDataTypeStr=uint32
  Divide12 : Product  Inputs=*/  OutDataTypeStr=double
  Divide13 : Product  Inputs=*/  OutDataTypeStr=uint32
  Float Const : Constant  Value=2  OutDataTypeStr=single
  Float Const6 : Constant  Value=0.5  OutDataTypeStr=single
  Subtract5 : Sum  Inputs=+-
  Out1 : Outport
  Out2 : Outport  Port=2
  wires:
  Float Const/1 -> [F_2]
  Divide12/1 -> Subtract5/1, Data Type Conversion5/1
  Divide13/1 -> Data Type Conversion9/1
  Float Const6/1 -> Divide13/2
  Data Type Conversion5/1 -> Out2/1, Subtract5/2
  [F_2] -> Divide12/2
  Subtract5/1 -> Divide13/1
  Data Type Conversion9/1 -> Out1/1
  In1/1 -> Divide12/1

== system ARINC429_DW/Decoder/De-serialize/Subsystem13 ==
  In1 : Inport
  Data Type Conversion5 : DataTypeConversion  OutDataTypeStr=uint32
  Data Type Conversion9 : DataTypeConversion  OutDataTypeStr=uint32
  Divide12 : Product  Inputs=*/  OutDataTypeStr=double
  Divide13 : Product  Inputs=*/  OutDataTypeStr=uint32
  Float Const : Constant  Value=2  OutDataTypeStr=single
  Float Const6 : Constant  Value=0.5  OutDataTypeStr=single
  Subtract5 : Sum  Inputs=+-
  Out1 : Outport
  Out2 : Outport  Port=2
  wires:
  Float Const/1 -> [F_2]
  Divide12/1 -> Subtract5/1, Data Type Conversion5/1
  Divide13/1 -> Data Type Conversion9/1
  Float Const6/1 -> Divide13/2
  Data Type Conversion5/1 -> Out2/1, Subtract5/2
  [F_2] -> Divide12/2
  Subtract5/1 -> Divide13/1
  Data Type Conversion9/1 -> Out1/1
  In1/1 -> Divide12/1

== system ARINC429_DW/Decoder/De-serialize/Subsystem14 ==
  In1 : Inport
  Data Type Conversion5 : DataTypeConversion  OutDataTypeStr=uint32
  Data Type Conversion9 : DataTypeConversion  OutDataTypeStr=uint32
  Divide12 : Product  Inputs=*/  OutDataTypeStr=double
  Divide13 : Product  Inputs=*/  OutDataTypeStr=uint32
  Float Const : Constant  Value=2  OutDataTypeStr=single
  Float Const6 : Constant  Value=0.5  OutDataTypeStr=single
  Subtract5 : Sum  Inputs=+-
  Out1 : Outport
  Out2 : Outport  Port=2
  wires:
  Float Const/1 -> [F_2]
  Divide12/1 -> Subtract5/1, Data Type Conversion5/1
  Divide13/1 -> Data Type Conversion9/1
  Float Const6/1 -> Divide13/2
  Data Type Conversion5/1 -> Out2/1, Subtract5/2
  [F_2] -> Divide12/2
  Subtract5/1 -> Divide13/1
  Data Type Conversion9/1 -> Out1/1
  In1/1 -> Divide12/1

== system ARINC429_DW/Decoder/De-serialize/Subsystem15 ==
  In1 : Inport
  Data Type Conversion5 : DataTypeConversion  OutDataTypeStr=uint32
  Data Type Conversion9 : DataTypeConversion  OutDataTypeStr=uint32
  Divide12 : Product  Inputs=*/  OutDataTypeStr=double
  Divide13 : Product  Inputs=*/  OutDataTypeStr=uint32
  Float Const : Constant  Value=2  OutDataTypeStr=single
  Float Const6 : Constant  Value=0.5  OutDataTypeStr=single
  Subtract5 : Sum  Inputs=+-
  Out1 : Outport
  Out2 : Outport  Port=2
  wires:
  Float Const/1 -> [F_2]
  Divide12/1 -> Subtract5/1, Data Type Conversion5/1
  Divide13/1 -> Data Type Conversion9/1
  Float Const6/1 -> Divide13/2
  Data Type Conversion5/1 -> Out2/1, Subtract5/2
  [F_2] -> Divide12/2
  Subtract5/1 -> Divide13/1
  Data Type Conversion9/1 -> Out1/1
  In1/1 -> Divide12/1

== system ARINC429_DW/Decoder/De-serialize/Subsystem16 ==
  In1 : Inport
  Data Type Conversion5 : DataTypeConversion  OutDataTypeStr=uint32
  Data Type Conversion9 : DataTypeConversion  OutDataTypeStr=uint32
  Divide12 : Product  Inputs=*/  OutDataTypeStr=double
  Divide13 : Product  Inputs=*/  OutDataTypeStr=uint32
  Float Const : Constant  Value=2  OutDataTypeStr=single
  Float Const6 : Constant  Value=0.5  OutDataTypeStr=single
  Subtract5 : Sum  Inputs=+-
  Out1 : Outport
  Out2 : Outport  Port=2
  wires:
  Float Const/1 -> [F_2]
  Divide12/1 -> Subtract5/1, Data Type Conversion5/1
  Divide13/1 -> Data Type Conversion9/1
  Float Const6/1 -> Divide13/2
  Data Type Conversion5/1 -> Out2/1, Subtract5/2
  [F_2] -> Divide12/2
  Subtract5/1 -> Divide13/1
  Data Type Conversion9/1 -> Out1/1
  In1/1 -> Divide12/1

== system ARINC429_DW/Decoder/De-serialize/Subsystem17 ==
  In1 : Inport
  Data Type Conversion5 : DataTypeConversion  OutDataTypeStr=uint32
  Data Type Conversion9 : DataTypeConversion  OutDataTypeStr=uint32
  Divide12 : Product  Inputs=*/  OutDataTypeStr=double
  Divide13 : Product  Inputs=*/  OutDataTypeStr=uint32
  Float Const : Constant  Value=2  OutDataTypeStr=single
  Float Const6 : Constant  Value=0.5  OutDataTypeStr=single
  Subtract5 : Sum  Inputs=+-
  Out1 : Outport
  Out2 : Outport  Port=2
  wires:
  Float Const/1 -> [F_2]
  Divide12/1 -> Subtract5/1, Data Type Conversion5/1
  Divide13/1 -> Data Type Conversion9/1
  Float Const6/1 -> Divide13/2
  Data Type Conversion5/1 -> Out2/1, Subtract5/2
  [F_2] -> Divide12/2
  Subtract5/1 -> Divide13/1
  Data Type Conversion9/1 -> Out1/1
  In1/1 -> Divide12/1

== system ARINC429_DW/Decoder/De-serialize/Subsystem18 ==
  In1 : Inport
  Data Type Conversion5 : DataTypeConversion  OutDataTypeStr=uint32
  Data Type Conversion9 : DataTypeConversion  OutDataTypeStr=uint32
  Divide12 : Product  Inputs=*/
  Divide13 : Product  Inputs=*/  OutDataTypeStr=uint32
  Float Const : Constant  Value=2  OutDataTypeStr=single
  Float Const6 : Constant  Value=0.5  OutDataTypeStr=single
  Subtract5 : Sum  Inputs=+-
  Out1 : Outport
  Out2 : Outport  Port=2
  wires:
  Float Const/1 -> [F_2]
  Divide12/1 -> Subtract5/1, Data Type Conversion5/1
  Divide13/1 -> Data Type Conversion9/1
  Float Const6/1 -> Divide13/2
  Data Type Conversion5/1 -> Out2/1, Subtract5/2
  [F_2] -> Divide12/2
  Subtract5/1 -> Divide13/1
  Data Type Conversion9/1 -> Out1/1
  In1/1 -> Divide12/1

== system ARINC429_DW/Decoder/De-serialize/Subsystem19 ==
  In1 : Inport
  Data Type Conversion5 : DataTypeConversion  OutDataTypeStr=uint32
  Data Type Conversion9 : DataTypeConversion  OutDataTypeStr=uint32
  Divide12 : Product  Inputs=*/
  Divide13 : Product  Inputs=*/  OutDataTypeStr=uint32
  Float Const : Constant  Value=2  OutDataTypeStr=single
  Float Const6 : Constant  Value=0.5  OutDataTypeStr=single
  Subtract5 : Sum  Inputs=+-
  Out1 : Outport
  Out2 : Outport  Port=2
  wires:
  Float Const/1 -> [F_2]
  Divide12/1 -> Subtract5/1, Data Type Conversion5/1
  Divide13/1 -> Data Type Conversion9/1
  Float Const6/1 -> Divide13/2
  Data Type Conversion5/1 -> Out2/1, Subtract5/2
  [F_2] -> Divide12/2
  Subtract5/1 -> Divide13/1
  Data Type Conversion9/1 -> Out1/1
  In1/1 -> Divide12/1

== system ARINC429_DW/Decoder/De-serialize/Subsystem2 ==
  In1 : Inport
  Data Type Conversion5 : DataTypeConversion  OutDataTypeStr=uint32
  Data Type Conversion9 : DataTypeConversion  OutDataTypeStr=uint32
  Divide12 : Product  Inputs=*/  OutDataTypeStr=double
  Divide13 : Product  Inputs=*/  OutDataTypeStr=uint32
  Float Const : Constant  Value=2  OutDataTypeStr=single
  Float Const6 : Constant  Value=0.5  OutDataTypeStr=single
  Subtract5 : Sum  Inputs=+-
  Out1 : Outport
  Out2 : Outport  Port=2
  wires:
  Float Const/1 -> [F_2]
  Divide12/1 -> Subtract5/1, Data Type Conversion5/1
  Divide13/1 -> Data Type Conversion9/1
  Float Const6/1 -> Divide13/2
  Data Type Conversion5/1 -> Out2/1, Subtract5/2
  [F_2] -> Divide12/2
  Subtract5/1 -> Divide13/1
  Data Type Conversion9/1 -> Out1/1
  In1/1 -> Divide12/1

== system ARINC429_DW/Decoder/De-serialize/Subsystem20 ==
  In1 : Inport
  Data Type Conversion5 : DataTypeConversion  OutDataTypeStr=uint32
  Data Type Conversion9 : DataTypeConversion  OutDataTypeStr=uint32
  Divide12 : Product  Inputs=*/
  Divide13 : Product  Inputs=*/  OutDataTypeStr=uint32
  Float Const : Constant  Value=2  OutDataTypeStr=single
  Float Const6 : Constant  Value=0.5  OutDataTypeStr=single
  Subtract5 : Sum  Inputs=+-
  Out1 : Outport
  Out2 : Outport  Port=2
  wires:
  Float Const/1 -> [F_2]
  Divide12/1 -> Subtract5/1, Data Type Conversion5/1
  Divide13/1 -> Data Type Conversion9/1
  Float Const6/1 -> Divide13/2
  Data Type Conversion5/1 -> Out2/1, Subtract5/2
  [F_2] -> Divide12/2
  Subtract5/1 -> Divide13/1
  Data Type Conversion9/1 -> Out1/1
  In1/1 -> Divide12/1

== system ARINC429_DW/Decoder/De-serialize/Subsystem21 ==
  In1 : Inport
  Data Type Conversion5 : DataTypeConversion  OutDataTypeStr=uint32
  Data Type Conversion9 : DataTypeConversion  OutDataTypeStr=uint32
  Divide12 : Product  Inputs=*/
  Divide13 : Product  Inputs=*/  OutDataTypeStr=uint32
  Float Const : Constant  Value=2  OutDataTypeStr=single
  Float Const6 : Constant  Value=0.5  OutDataTypeStr=single
  Subtract5 : Sum  Inputs=+-
  Out1 : Outport
  Out2 : Outport  Port=2
  wires:
  Float Const/1 -> [F_2]
  Divide12/1 -> Subtract5/1, Data Type Conversion5/1
  Divide13/1 -> Data Type Conversion9/1
  Float Const6/1 -> Divide13/2
  Data Type Conversion5/1 -> Out2/1, Subtract5/2
  [F_2] -> Divide12/2
  Subtract5/1 -> Divide13/1
  Data Type Conversion9/1 -> Out1/1
  In1/1 -> Divide12/1

== system ARINC429_DW/Decoder/De-serialize/Subsystem22 ==
  In1 : Inport
  Data Type Conversion5 : DataTypeConversion  OutDataTypeStr=uint32
  Data Type Conversion9 : DataTypeConversion  OutDataTypeStr=uint32
  Divide12 : Product  Inputs=*/
  Divide13 : Product  Inputs=*/  OutDataTypeStr=uint32
  Float Const : Constant  Value=2  OutDataTypeStr=single
  Float Const6 : Constant  Value=0.5  OutDataTypeStr=single
  Subtract5 : Sum  Inputs=+-
  Out1 : Outport
  Out2 : Outport  Port=2
  wires:
  Float Const/1 -> [F_2]
  Divide12/1 -> Subtract5/1, Data Type Conversion5/1
  Divide13/1 -> Data Type Conversion9/1
  Float Const6/1 -> Divide13/2
  Data Type Conversion5/1 -> Out2/1, Subtract5/2
  [F_2] -> Divide12/2
  Subtract5/1 -> Divide13/1
  Data Type Conversion9/1 -> Out1/1
  In1/1 -> Divide12/1

== system ARINC429_DW/Decoder/De-serialize/Subsystem23 ==
  In1 : Inport
  Data Type Conversion5 : DataTypeConversion  OutDataTypeStr=uint32
  Data Type Conversion9 : DataTypeConversion  OutDataTypeStr=uint32
  Divide12 : Product  Inputs=*/
  Divide13 : Product  Inputs=*/  OutDataTypeStr=uint32
  Float Const : Constant  Value=2  OutDataTypeStr=single
  Float Const6 : Constant  Value=0.5  OutDataTypeStr=single
  Subtract5 : Sum  Inputs=+-
  Out1 : Outport
  Out2 : Outport  Port=2
  wires:
  Float Const/1 -> [F_2]
  Divide12/1 -> Subtract5/1, Data Type Conversion5/1
  Divide13/1 -> Data Type Conversion9/1
  Float Const6/1 -> Divide13/2
  Data Type Conversion5/1 -> Out2/1, Subtract5/2
  [F_2] -> Divide12/2
  Subtract5/1 -> Divide13/1
  Data Type Conversion9/1 -> Out1/1
  In1/1 -> Divide12/1

== system ARINC429_DW/Decoder/De-serialize/Subsystem24 ==
  In1 : Inport
  Data Type Conversion5 : DataTypeConversion  OutDataTypeStr=uint32
  Data Type Conversion9 : DataTypeConversion  OutDataTypeStr=uint32
  Divide12 : Product  Inputs=*/
  Divide13 : Product  Inputs=*/  OutDataTypeStr=uint32
  Float Const : Constant  Value=2  OutDataTypeStr=single
  Float Const6 : Constant  Value=0.5  OutDataTypeStr=single
  Subtract5 : Sum  Inputs=+-
  Out1 : Outport
  Out2 : Outport  Port=2
  wires:
  Float Const/1 -> [F_2]
  Divide12/1 -> Subtract5/1, Data Type Conversion5/1
  Divide13/1 -> Data Type Conversion9/1
  Float Const6/1 -> Divide13/2
  Data Type Conversion5/1 -> Out2/1, Subtract5/2
  [F_2] -> Divide12/2
  Subtract5/1 -> Divide13/1
  Data Type Conversion9/1 -> Out1/1
  In1/1 -> Divide12/1

== system ARINC429_DW/Decoder/De-serialize/Subsystem25 ==
  In1 : Inport
  Data Type Conversion5 : DataTypeConversion  OutDataTypeStr=uint32
  Data Type Conversion9 : DataTypeConversion  OutDataTypeStr=uint32
  Divide12 : Product  Inputs=*/
  Divide13 : Product  Inputs=*/  OutDataTypeStr=uint32
  Float Const : Constant  Value=2  OutDataTypeStr=single
  Float Const6 : Constant  Value=0.5  OutDataTypeStr=single
  Subtract5 : Sum  Inputs=+-
  Out1 : Outport
  Out2 : Outport  Port=2
  wires:
  Float Const/1 -> [F_2]
  Divide12/1 -> Subtract5/1, Data Type Conversion5/1
  Divide13/1 -> Data Type Conversion9/1
  Float Const6/1 -> Divide13/2
  Data Type Conversion5/1 -> Out2/1, Subtract5/2
  [F_2] -> Divide12/2
  Subtract5/1 -> Divide13/1
  Data Type Conversion9/1 -> Out1/1
  In1/1 -> Divide12/1

== system ARINC429_DW/Decoder/De-serialize/Subsystem26 ==
  In1 : Inport
  Data Type Conversion5 : DataTypeConversion  OutDataTypeStr=uint32
  Data Type Conversion9 : DataTypeConversion  OutDataTypeStr=uint32
  Divide12 : Product  Inputs=*/
  Divide13 : Product  Inputs=*/  OutDataTypeStr=uint32
  Float Const : Constant  Value=2  OutDataTypeStr=single
  Float Const6 : Constant  Value=0.5  OutDataTypeStr=single
  Subtract5 : Sum  Inputs=+-
  Out1 : Outport
  Out2 : Outport  Port=2
  wires:
  Float Const/1 -> [F_2]
  Divide12/1 -> Subtract5/1, Data Type Conversion5/1
  Divide13/1 -> Data Type Conversion9/1
  Float Const6/1 -> Divide13/2
  Data Type Conversion5/1 -> Out2/1, Subtract5/2
  [F_2] -> Divide12/2
  Subtract5/1 -> Divide13/1
  Data Type Conversion9/1 -> Out1/1
  In1/1 -> Divide12/1

== system ARINC429_DW/Decoder/De-serialize/Subsystem27 ==
  In1 : Inport
  Data Type Conversion5 : DataTypeConversion  OutDataTypeStr=uint32
  Data Type Conversion9 : DataTypeConversion  OutDataTypeStr=uint32
  Divide12 : Product  Inputs=*/
  Divide13 : Product  Inputs=*/  OutDataTypeStr=uint32
  Float Const : Constant  Value=2  OutDataTypeStr=single
  Float Const6 : Constant  Value=0.5  OutDataTypeStr=single
  Subtract5 : Sum  Inputs=+-
  Out1 : Outport
  Out2 : Outport  Port=2
  wires:
  Float Const/1 -> [F_2]
  Divide12/1 -> Subtract5/1, Data Type Conversion5/1
  Divide13/1 -> Data Type Conversion9/1
  Float Const6/1 -> Divide13/2
  Data Type Conversion5/1 -> Out2/1, Subtract5/2
  [F_2] -> Divide12/2
  Subtract5/1 -> Divide13/1
  Data Type Conversion9/1 -> Out1/1
  In1/1 -> Divide12/1

== system ARINC429_DW/Decoder/De-serialize/Subsystem28 ==
  In1 : Inport
  Data Type Conversion5 : DataTypeConversion  OutDataTypeStr=uint32
  Data Type Conversion9 : DataTypeConversion  OutDataTypeStr=uint32
  Divide12 : Product  Inputs=*/
  Divide13 : Product  Inputs=*/  OutDataTypeStr=uint32
  Float Const : Constant  Value=2  OutDataTypeStr=single
  Float Const6 : Constant  Value=0.5  OutDataTypeStr=single
  Subtract5 : Sum  Inputs=+-
  Out1 : Outport
  Out2 : Outport  Port=2
  wires:
  Float Const/1 -> [F_2]
  Divide12/1 -> Subtract5/1, Data Type Conversion5/1
  Divide13/1 -> Data Type Conversion9/1
  Float Const6/1 -> Divide13/2
  Data Type Conversion5/1 -> Out2/1, Subtract5/2
  [F_2] -> Divide12/2
  Subtract5/1 -> Divide13/1
  Data Type Conversion9/1 -> Out1/1
  In1/1 -> Divide12/1

== system ARINC429_DW/Decoder/De-serialize/Subsystem29 ==
  In1 : Inport
  Data Type Conversion5 : DataTypeConversion  OutDataTypeStr=uint32
  Data Type Conversion9 : DataTypeConversion  OutDataTypeStr=uint32
  Divide12 : Product  Inputs=*/
  Divide13 : Product  Inputs=*/  OutDataTypeStr=uint32
  Float Const : Constant  Value=2  OutDataTypeStr=single
  Float Const6 : Constant  Value=0.5  OutDataTypeStr=single
  Subtract5 : Sum  Inputs=+-
  Out1 : Outport
  Out2 : Outport  Port=2
  wires:
  Float Const/1 -> [F_2]
  Divide12/1 -> Subtract5/1, Data Type Conversion5/1
  Divide13/1 -> Data Type Conversion9/1
  Float Const6/1 -> Divide13/2
  Data Type Conversion5/1 -> Out2/1, Subtract5/2
  [F_2] -> Divide12/2
  Subtract5/1 -> Divide13/1
  Data Type Conversion9/1 -> Out1/1
  In1/1 -> Divide12/1

== system ARINC429_DW/Decoder/De-serialize/Subsystem3 ==
  In1 : Inport
  Data Type Conversion5 : DataTypeConversion  OutDataTypeStr=uint32
  Data Type Conversion9 : DataTypeConversion  OutDataTypeStr=uint32
  Divide12 : Product  Inputs=*/  OutDataTypeStr=double
  Divide13 : Product  Inputs=*/
  Float Const : Constant  Value=2  OutDataTypeStr=single
  Float Const6 : Constant  Value=0.5  OutDataTypeStr=single
  Subtract5 : Sum  Inputs=+-
  Out1 : Outport
  Out2 : Outport  Port=2
  wires:
  Float Const/1 -> [F_2]
  Divide12/1 -> Subtract5/1, Data Type Conversion5/1
  Divide13/1 -> Data Type Conversion9/1
  Float Const6/1 -> Divide13/2
  Data Type Conversion5/1 -> Out2/1, Subtract5/2
  In1/1 -> Divide12/1
  [F_2] -> Divide12/2
  Subtract5/1 -> Divide13/1
  Data Type Conversion9/1 -> Out1/1

== system ARINC429_DW/Decoder/De-serialize/Subsystem30 ==
  In1 : Inport
  Data Type Conversion5 : DataTypeConversion  OutDataTypeStr=uint32
  Data Type Conversion9 : DataTypeConversion  OutDataTypeStr=uint32
  Divide12 : Product  Inputs=*/
  Divide13 : Product  Inputs=*/  OutDataTypeStr=uint32
  Float Const : Constant  Value=2  OutDataTypeStr=single
  Float Const6 : Constant  Value=0.5  OutDataTypeStr=single
  Subtract5 : Sum  Inputs=+-
  Out1 : Outport
  Out2 : Outport  Port=2
  wires:
  Float Const/1 -> [F_2]
  Divide12/1 -> Subtract5/1, Data Type Conversion5/1
  Divide13/1 -> Data Type Conversion9/1
  Float Const6/1 -> Divide13/2
  Data Type Conversion5/1 -> Out2/1, Subtract5/2
  [F_2] -> Divide12/2
  Subtract5/1 -> Divide13/1
  Data Type Conversion9/1 -> Out1/1
  In1/1 -> Divide12/1

== system ARINC429_DW/Decoder/De-serialize/Subsystem31 ==
  In1 : Inport
  Data Type Conversion5 : DataTypeConversion  OutDataTypeStr=uint32
  Data Type Conversion9 : DataTypeConversion  OutDataTypeStr=uint32
  Divide12 : Product  Inputs=*/
  Divide13 : Product  Inputs=*/  OutDataTypeStr=uint32
  Float Const : Constant  Value=2  OutDataTypeStr=single
  Float Const6 : Constant  Value=0.5  OutDataTypeStr=single
  Subtract5 : Sum  Inputs=+-
  Out1 : Outport
  Out2 : Outport  Port=2
  wires:
  Float Const/1 -> [F_2]
  Divide12/1 -> Subtract5/1, Data Type Conversion5/1
  Divide13/1 -> Data Type Conversion9/1
  Float Const6/1 -> Divide13/2
  Data Type Conversion5/1 -> Out2/1, Subtract5/2
  [F_2] -> Divide12/2
  Subtract5/1 -> Divide13/1
  Data Type Conversion9/1 -> Out1/1
  In1/1 -> Divide12/1

== system ARINC429_DW/Decoder/De-serialize/Subsystem32 ==
  In1 : Inport
  Data Type Conversion5 : DataTypeConversion  OutDataTypeStr=uint32
  Data Type Conversion9 : DataTypeConversion  OutDataTypeStr=uint32
  Divide12 : Product  Inputs=*/
  Divide13 : Product  Inputs=*/  OutDataTypeStr=uint32
  Float Const : Constant  Value=2  OutDataTypeStr=single
  Float Const6 : Constant  Value=0.5  OutDataTypeStr=single
  Subtract5 : Sum  Inputs=+-
  Out1 : Outport
  Out2 : Outport  Port=2
  wires:
  Float Const/1 -> [F_2]
  Divide12/1 -> Subtract5/1, Data Type Conversion5/1
  Divide13/1 -> Data Type Conversion9/1
  Float Const6/1 -> Divide13/2
  Data Type Conversion5/1 -> Out2/1, Subtract5/2
  [F_2] -> Divide12/2
  Subtract5/1 -> Divide13/1
  Data Type Conversion9/1 -> Out1/1
  In1/1 -> Divide12/1

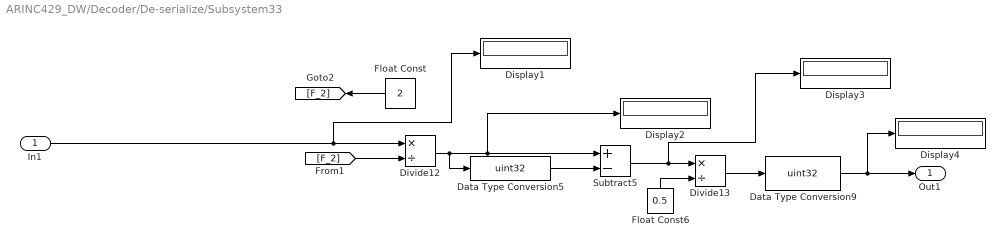
== system ARINC429_DW/Decoder/De-serialize/Subsystem33 ==
  In1 : Inport
  Data Type Conversion5 : DataTypeConversion  OutDataTypeStr=uint32
  Data Type Conversion9 : DataTypeConversion  OutDataTypeStr=uint32
  Display{1..4} (4 alike) : Display
      settings: Format=decimal (Stored Integer)
  Divide12 : Product  Inputs=*/  OutDataTypeStr=double
  Divide13 : Product  Inputs=*/  OutDataTypeStr=uint32
  Float Const : Constant  Value=2  OutDataTypeStr=single
  Float Const6 : Constant  Value=0.5  OutDataTypeStr=single
  Subtract5 : Sum  Inputs=+-
  Out1 : Outport
  wires:
  Float Const/1 -> [F_2]
  Divide12/1 -> Display2/1, Subtract5/1, Data Type Conversion5/1
  Divide13/1 -> Data Type Conversion9/1
  Float Const6/1 -> Divide13/2
  Data Type Conversion5/1 -> Subtract5/2
  [F_2] -> Divide12/2
  Subtract5/1 -> Display3/1, Divide13/1
  Data Type Conversion9/1 -> Display4/1, Out1/1
  In1/1 -> Display1/1, Divide12/1

== system ARINC429_DW/Decoder/De-serialize/Subsystem4 ==
  In1 : Inport
  Data Type Conversion5 : DataTypeConversion  OutDataTypeStr=uint32
  Data Type Conversion9 : DataTypeConversion  OutDataTypeStr=uint32
  Divide12 : Product  Inputs=*/  OutDataTypeStr=double
  Divide13 : Product  Inputs=*/  OutDataTypeStr=uint32
  Float Const : Constant  Value=2  OutDataTypeStr=single
  Float Const6 : Constant  Value=0.5  OutDataTypeStr=single
  Subtract5 : Sum  Inputs=+-
  Out1 : Outport
  Out2 : Outport  Port=2
  wires:
  Float Const/1 -> [F_2]
  Divide12/1 -> Subtract5/1, Data Type Conversion5/1
  Divide13/1 -> Data Type Conversion9/1
  Float Const6/1 -> Divide13/2
  Data Type Conversion5/1 -> Out2/1, Subtract5/2
  [F_2] -> Divide12/2
  Subtract5/1 -> Divide13/1
  Data Type Conversion9/1 -> Out1/1
  In1/1 -> Divide12/1

== system ARINC429_DW/Decoder/De-serialize/Subsystem7 ==
  In1 : Inport
  Data Type Conversion5 : DataTypeConversion  OutDataTypeStr=uint32
  Data Type Conversion9 : DataTypeConversion  OutDataTypeStr=uint32
  Divide12 : Product  Inputs=*/  OutDataTypeStr=double
  Divide13 : Product  Inputs=*/  OutDataTypeStr=uint32
  Float Const : Constant  Value=2  OutDataTypeStr=single
  Float Const6 : Constant  Value=0.5  OutDataTypeStr=single
  Subtract5 : Sum  Inputs=+-
  Out1 : Outport
  Out2 : Outport  Port=2
  wires:
  Float Const/1 -> [F_2]
  Divide12/1 -> Subtract5/1, Data Type Conversion5/1
  Divide13/1 -> Data Type Conversion9/1
  Float Const6/1 -> Divide13/2
  Data Type Conversion5/1 -> Out2/1, Subtract5/2
  [F_2] -> Divide12/2
  Subtract5/1 -> Divide13/1
  Data Type Conversion9/1 -> Out1/1
  In1/1 -> Divide12/1

== system ARINC429_DW/Decoder/De-serialize/Subsystem8 ==
  In1 : Inport
  Data Type Conversion5 : DataTypeConversion  OutDataTypeStr=uint32
  Data Type Conversion9 : DataTypeConversion  OutDataTypeStr=uint32
  Divide12 : Product  Inputs=*/  OutDataTypeStr=double
  Divide13 : Product  Inputs=*/  OutDataTypeStr=uint32
  Float Const : Constant  Value=2  OutDataTypeStr=single
  Float Const6 : Constant  Value=0.5  OutDataTypeStr=single
  Subtract5 : Sum  Inputs=+-
  Out1 : Outport
  Out2 : Outport  Port=2
  wires:
  Float Const/1 -> [F_2]
  Divide12/1 -> Subtract5/1, Data Type Conversion5/1
  Divide13/1 -> Data Type Conversion9/1
  Float Const6/1 -> Divide13/2
  Data Type Conversion5/1 -> Out2/1, Subtract5/2
  [F_2] -> Divide12/2
  Subtract5/1 -> Divide13/1
  Data Type Conversion9/1 -> Out1/1
  In1/1 -> Divide12/1

== system ARINC429_DW/Decoder/De-serialize/Subsystem9 ==
  In1 : Inport
  Data Type Conversion5 : DataTypeConversion  OutDataTypeStr=uint32
  Data Type Conversion9 : DataTypeConversion  OutDataTypeStr=uint32
  Divide12 : Product  Inputs=*/  OutDataTypeStr=double
  Divide13 : Product  Inputs=*/  OutDataTypeStr=uint32
  Float Const : Constant  Value=2  OutDataTypeStr=single
  Float Const6 : Constant  Value=0.5  OutDataTypeStr=single
  Subtract5 : Sum  Inputs=+-
  Out1 : Outport
  Out2 : Outport  Port=2
  wires:
  Float Const/1 -> [F_2]
  Divide12/1 -> Subtract5/1, Data Type Conversion5/1
  Divide13/1 -> Data Type Conversion9/1
  Float Const6/1 -> Divide13/2
  Data Type Conversion5/1 -> Out2/1, Subtract5/2
  [F_2] -> Divide12/2
  Subtract5/1 -> Divide13/1
  Data Type Conversion9/1 -> Out1/1
  In1/1 -> Divide12/1
